simulink model "Induction_Machine_Model"  (Simulink 7.5)
settings: Solver=ode45  StartTime=0.0  StopTime=10.0  RelTol=1e-3
settings Model: Creator=CN  LastModifiedBy=pradhyumna
settings DebuggingCC: StrictBusMsg=Warning

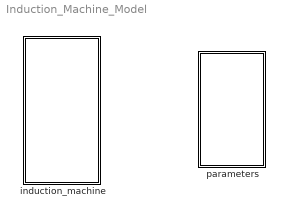
== system Induction_Machine_Model ==
  induction_machine : Subsystem
  parameters : Subsystem

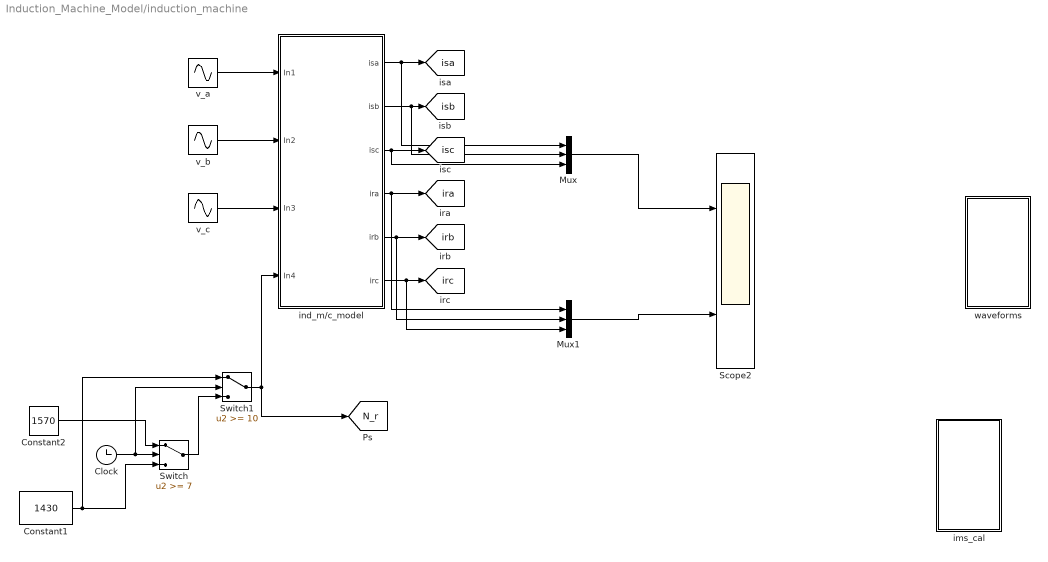
== system Induction_Machine_Model/induction_machine ==
  Clock : Clock
      settings: Decimation=10
  Constant1 : Constant  Value=1430  OutDataType=sfix(16)  OutScaling=2^0
  Constant2 : Constant  Value=1570  OutDataType=sfix(16)  OutScaling=2^0
  Mux : Mux  Inputs=3
  Mux1 : Mux  Inputs=3
  Scope2 : Scope  NumInputPorts=2
      settings: TimeRange=4.5  YMin=-30~-30  YMax=30~30  SampleInput=on  SampleTime=0.00001
  Switch : Switch  Threshold=7
  Switch1 : Switch  Threshold=10
  ims_cal : Subsystem
  ind_m/c_model : Subsystem
  v_a : Sin  Amplitude=239.6*sqrt(2)  Bias=0  Frequency=2*pi*50  Phase=0  Samples=10  SampleTime=0  Offset=0
  v_b : Sin  Amplitude=239.6*sqrt(2)  Bias=0  Frequency=2*pi*50  Phase=-2*pi/3  Samples=10  SampleTime=0  Offset=0
  v_c : Sin  Amplitude=239.6*sqrt(2)  Bias=0  Frequency=2*pi*50  Phase=-4*pi/3  Samples=10  SampleTime=0  Offset=0
  waveforms : Subsystem
  tag scope: N_r=global, ira=global, irb=global, irc=global, isa=global, isb=global, isc=global
  wires:
  ind_m/c_model/6(irc) -> [irc], Mux1/3
  ind_m/c_model/5(irb) -> [irb], Mux1/2
  ind_m/c_model/4(ira) -> [ira], Mux1/1
  ind_m/c_model/3(isc) -> [isc], Mux/3
  ind_m/c_model/2(isb) -> [isb], Mux/2
  ind_m/c_model/1(isa) -> [isa], Mux/1
  v_c/1 -> ind_m/c_model/3(In3)
  v_b/1 -> ind_m/c_model/2(In2)
  v_a/1 -> ind_m/c_model/1(In1)
  Mux/1 -> Scope2/1
  Mux1/1 -> Scope2/2
  Clock/1 -> Switch/2, Switch1/2
  Constant2/1 -> Switch/1
  Constant1/1 -> Switch/3, Switch1/1
  Switch/1 -> Switch1/3
  Switch1/1 -> ind_m/c_model/4(In4), [N_r]

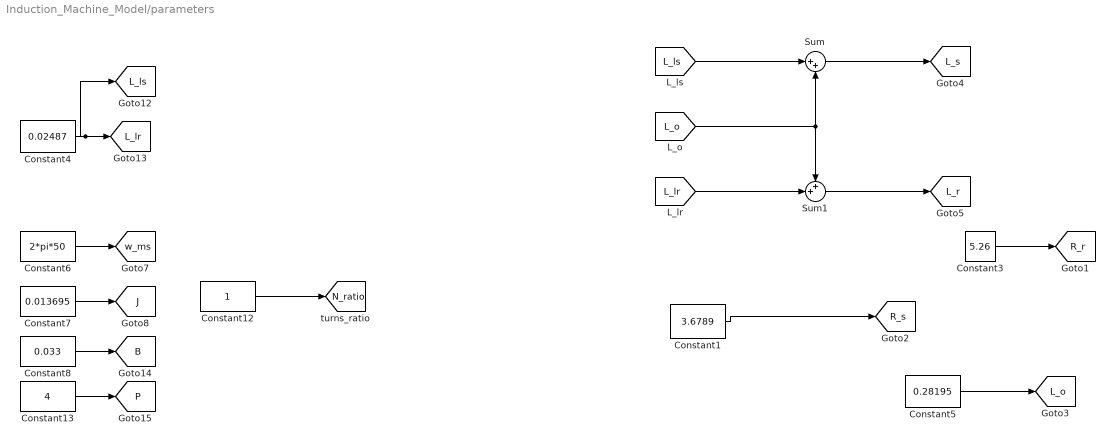
== system Induction_Machine_Model/parameters ==
  Constant1 : Constant  Value=3.6789  OutDataType=sfix(16)  OutScaling=2^0
  Constant12 : Constant  OutDataType=sfix(16)  OutScaling=2^0
  Constant13 : Constant  Value=4  OutDataType=sfix(16)  OutScaling=2^0
  Constant3 : Constant  Value=5.26  OutDataType=sfix(16)  OutScaling=2^0
  Constant4 : Constant  Value=0.02487  OutDataType=sfix(16)  OutScaling=2^0
  Constant5 : Constant  Value=0.28195  OutDataType=sfix(16)  OutScaling=2^0
  Constant6 : Constant  Value=2*pi*50  OutDataType=sfix(16)  OutScaling=2^0
  Constant7 : Constant  Value=0.013695  OutDataType=sfix(16)  OutScaling=2^0
  Constant8 : Constant  Value=0.033  OutDataType=sfix(16)  OutScaling=2^0
  Sum : Sum  Inputs=|++  OutDataType=sfix(16)  OutScaling=2^0
  Sum1 : Sum  Inputs=++|  OutDataType=sfix(16)  OutScaling=2^0
  tag scope: B=global, J=global, L_lr=global, L_ls=global, L_o=global, L_r=global, L_s=global, N_ratio=global, P=global, R_r=global, R_s=global, w_ms=global
  wires:
  Constant4/1 -> [L_lr], [L_ls]
  Constant6/1 -> [w_ms]
  Constant7/1 -> [J]
  Constant8/1 -> [B]
  Constant13/1 -> [P]
  Constant12/1 -> [N_ratio]
  [L_lr] -> Sum1/2
  [L_ls] -> Sum/1
  [L_o] -> Sum/2, Sum1/1
  Sum/1 -> [L_s]
  Sum1/1 -> [L_r]
  Constant3/1 -> [R_r]
  Constant5/1 -> [L_o]
  Constant1/1 -> [R_s]

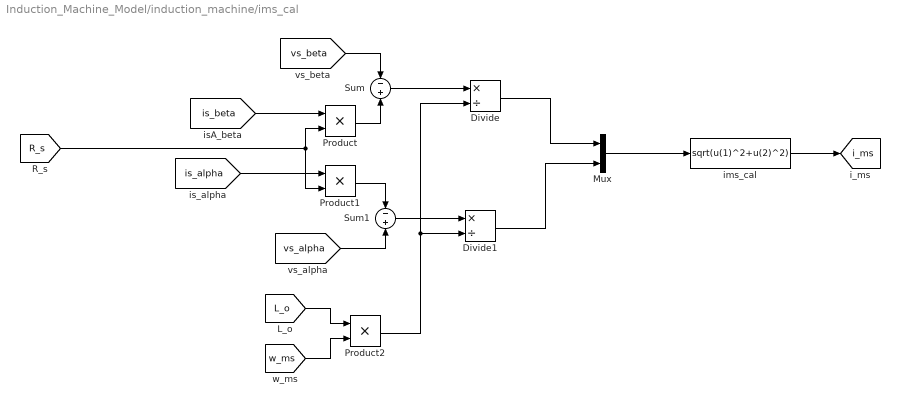
== system Induction_Machine_Model/induction_machine/ims_cal ==
  Divide : Product  Inputs=*/  OutDataType=sfix(16)  OutScaling=2^-10
  Divide1 : Product  Inputs=*/  OutDataType=sfix(16)  OutScaling=2^-10
  Mux : Mux  Inputs=2
  Product : Product  OutDataType=sfix(16)  OutScaling=2^0  RndMeth=Zero
  Product1 : Product  OutDataType=sfix(16)  OutScaling=2^0  RndMeth=Zero
  Product2 : Product  OutDataType=sfix(16)  OutScaling=2^0  RndMeth=Zero
  Sum : Sum  Inputs=-+  OutDataType=sfix(16)  OutScaling=2^0
  Sum1 : Sum  Inputs=-+  OutDataType=sfix(16)  OutScaling=2^0
  ims_cal : Fcn  Expr=sqrt(u(1)^2+u(2)^2)
  tag scope: i_ms=global
  wires:
  [is_beta] -> Product/1
  [is_alpha] -> Product1/1
  [R_s] -> Product/2, Product1/2
  [vs_beta] -> Sum/1
  Product/1 -> Sum/2
  Product1/1 -> Sum1/1
  [vs_alpha] -> Sum1/2
  [L_o] -> Product2/1
  [w_ms] -> Product2/2
  Sum/1 -> Divide/1
  Sum1/1 -> Divide1/1
  Product2/1 -> Divide/2, Divide1/2
  Divide/1 -> Mux/1
  Divide1/1 -> Mux/2
  Mux/1 -> ims_cal/1
  ims_cal/1 -> [i_ms]

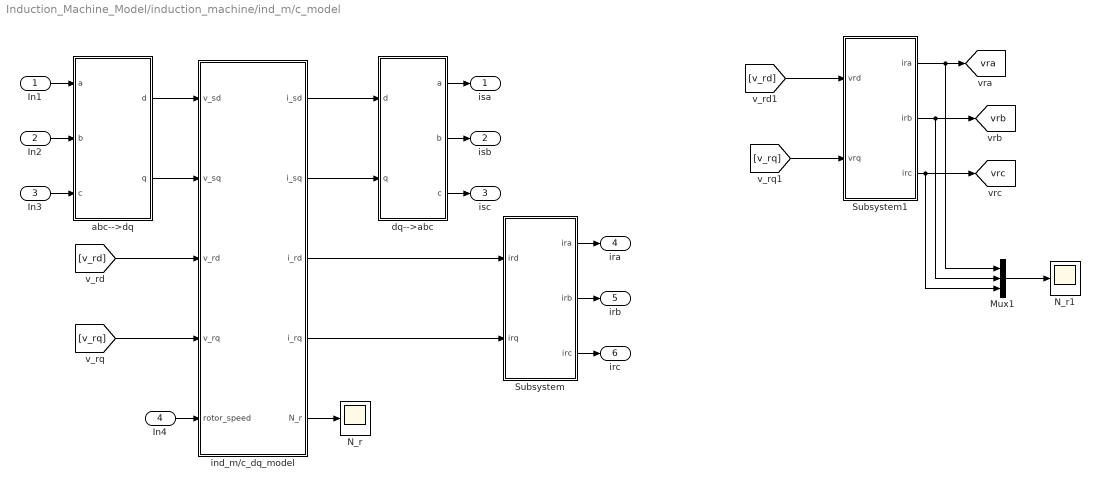
== system Induction_Machine_Model/induction_machine/ind_m/c_model ==
  In1 : Inport  OutDataType=sfix(16)  OutScaling=2^0
  In2 : Inport  Port=2  OutDataType=sfix(16)  OutScaling=2^0
  In3 : Inport  Port=3  OutDataType=sfix(16)  OutScaling=2^0
  In4 : Inport  Port=4  OutDataType=sfix(16)  OutScaling=2^0
  Mux1 : Mux  Inputs=3
  N_r : Scope
      settings: TimeRange=3  YMin=-7460  YMax=-7390  SaveName=ScopeData5  SampleInput=on  SampleTime=0.0001
  N_r1 : Scope
      settings: TimeRange=3  YMin=-7460  YMax=-7390  SaveName=ScopeData2  SampleInput=on  SampleTime=0.0001
  Subsystem : Subsystem
  Subsystem1 : Subsystem
  abc-->dq : Subsystem
  dq-->abc : Subsystem
  ind_m/c_dq_model : Subsystem
  isa : Outport  OutDataType=sfix(16)  OutScaling=2^0
  isb : Outport  Port=2  OutDataType=sfix(16)  OutScaling=2^0
  isc : Outport  Port=3  OutDataType=sfix(16)  OutScaling=2^0
  ira : Outport  Port=4  OutDataType=sfix(16)  OutScaling=2^0
  irb : Outport  Port=5  OutDataType=sfix(16)  OutScaling=2^0
  irc : Outport  Port=6  OutDataType=sfix(16)  OutScaling=2^0
  tag scope: vra=global, vrb=global, vrc=global
  wires:
  ind_m/c_dq_model/1(i_sd) -> dq-->abc/1(d)
  ind_m/c_dq_model/2(i_sq) -> dq-->abc/2(q)
  ind_m/c_dq_model/5(N_r) -> N_r/1
  abc-->dq/2(q) -> ind_m/c_dq_model/2(v_sq)
  abc-->dq/1(d) -> ind_m/c_dq_model/1(v_sd)
  ind_m/c_dq_model/3(i_rd) -> Subsystem/1(ird)
  ind_m/c_dq_model/4(i_rq) -> Subsystem/2(irq)
  In1/1 -> abc-->dq/1(a)
  dq-->abc/1(a) -> isa/1
  In2/1 -> abc-->dq/2(b)
  dq-->abc/2(b) -> isb/1
  In3/1 -> abc-->dq/3(c)
  dq-->abc/3(c) -> isc/1
  Subsystem/1(ira) -> ira/1
  Subsystem/2(irb) -> irb/1
  Subsystem/3(irc) -> irc/1
  In4/1 -> ind_m/c_dq_model/5(rotor_speed)
  [v_rd] -> ind_m/c_dq_model/3(v_rd)
  [v_rq] -> ind_m/c_dq_model/4(v_rq)
  [v_rd] -> Subsystem1/1(vrd)
  [v_rq] -> Subsystem1/2(vrq)
  Subsystem1/1(ira) -> [vra], Mux1/1
  Subsystem1/2(irb) -> [vrb], Mux1/2
  Subsystem1/3(irc) -> [vrc], Mux1/3
  Mux1/1 -> N_r1/1

== system Induction_Machine_Model/induction_machine/waveforms ==
  Mux : Mux  Inputs=3
  Mux1 : Mux  Inputs=3
  Mux2 : Mux  Inputs=3
  N_r : Scope  NumInputPorts=3
      settings: TimeRange=3  YMin=-7460~-5~-5  YMax=-7390~5~5  SampleInput=on  SampleTime=0.00001
  wires:
  [vsa] -> Mux/1
  [vsb] -> Mux/2
  [vsc] -> Mux/3
  [isa] -> Mux1/1
  [isb] -> Mux1/2
  [isc] -> Mux1/3
  [ira] -> Mux2/1
  [irb] -> Mux2/2
  [irc] -> Mux2/3
  Mux/1 -> N_r/1
  Mux1/1 -> N_r/2
  Mux2/1 -> N_r/3

== system Induction_Machine_Model/induction_machine/ind_m/c_model/Subsystem ==
  ird : Inport  OutDataType=sfix(16)  OutScaling=2^0
  irq : Inport  Port=2  OutDataType=sfix(16)  OutScaling=2^0
  ab-->abc : Subsystem
  dq-->ab : Subsystem
  ira : Outport  OutDataType=sfix(16)  OutScaling=2^0
  irb : Outport  Port=2  OutDataType=sfix(16)  OutScaling=2^0
  irc : Outport  Port=3  OutDataType=sfix(16)  OutScaling=2^0
  wires:
  dq-->ab/1(ir_a) -> ab-->abc/1(ir_a)
  dq-->ab/2(ir_b) -> ab-->abc/2(ir_b)
  ab-->abc/1(a) -> ira/1
  ird/1 -> dq-->ab/1(ird)
  ab-->abc/2(b) -> irb/1
  irq/1 -> dq-->ab/2(irq)
  ab-->abc/3(c) -> irc/1

== system Induction_Machine_Model/induction_machine/ind_m/c_model/Subsystem1 ==
  vrd : Inport  OutDataType=sfix(16)  OutScaling=2^0
  vrq : Inport  Port=2  OutDataType=sfix(16)  OutScaling=2^0
  ab-->abc : Subsystem
  dq-->ab : Subsystem
  ira : Outport  OutDataType=sfix(16)  OutScaling=2^0
  irb : Outport  Port=2  OutDataType=sfix(16)  OutScaling=2^0
  irc : Outport  Port=3  OutDataType=sfix(16)  OutScaling=2^0
  wires:
  ab-->abc/3(c) -> irc/1
  vrq/1 -> dq-->ab/2(vrq)
  ab-->abc/2(b) -> irb/1
  vrd/1 -> dq-->ab/1(vrd)
  ab-->abc/1(a) -> ira/1
  dq-->ab/2(ir_b) -> ab-->abc/2(ir_b)
  dq-->ab/1(ir_a) -> ab-->abc/1(ir_a)

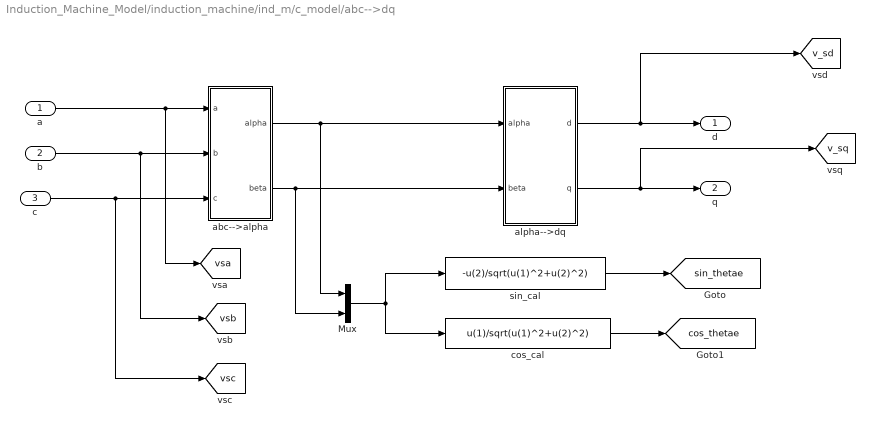
== system Induction_Machine_Model/induction_machine/ind_m/c_model/abc-->dq ==
  a : Inport  OutDataType=sfix(16)  OutScaling=2^0
  b : Inport  Port=2  OutDataType=sfix(16)  OutScaling=2^0
  c : Inport  Port=3  OutDataType=sfix(16)  OutScaling=2^0
  Mux : Mux  Inputs=2
  abc-->alpha : Subsystem
  alpha-->dq : Subsystem
  cos_cal : Fcn  Expr=u(1)/sqrt(u(1)^2+u(2)^2)
  sin_cal : Fcn  Expr=-u(2)/sqrt(u(1)^2+u(2)^2)
  d : Outport  OutDataType=sfix(16)  OutScaling=2^0
  q : Outport  Port=2  OutDataType=sfix(16)  OutScaling=2^0
  tag scope: cos_thetae=global, sin_thetae=global, v_sd=global, v_sq=global, vsa=global, vsb=global, vsc=global
  wires:
  abc-->alpha/1(alpha) -> alpha-->dq/1(alpha), Mux/1
  abc-->alpha/2(beta) -> alpha-->dq/2(beta), Mux/2
  a/1 -> abc-->alpha/1(a), [vsa]
  alpha-->dq/1(d) -> d/1, [v_sd]
  b/1 -> abc-->alpha/2(b), [vsb]
  alpha-->dq/2(q) -> q/1, [v_sq]
  c/1 -> abc-->alpha/3(c), [vsc]
  Mux/1 -> sin_cal/1, cos_cal/1
  sin_cal/1 -> [sin_thetae]
  cos_cal/1 -> [cos_thetae]

== system Induction_Machine_Model/induction_machine/ind_m/c_model/dq-->abc ==
  d : Inport  OutDataType=sfix(16)  OutScaling=2^0
  q : Inport  Port=2  OutDataType=sfix(16)  OutScaling=2^0
  alpha-->abc : Subsystem
  dq-->alpha : Subsystem
  a : Outport  OutDataType=sfix(16)  OutScaling=2^0
  b : Outport  Port=2  OutDataType=sfix(16)  OutScaling=2^0
  c : Outport  Port=3  OutDataType=sfix(16)  OutScaling=2^0
  wires:
  dq-->alpha/1(alpha) -> alpha-->abc/1(alpha)
  dq-->alpha/2(beta) -> alpha-->abc/2(beta)
  alpha-->abc/1(a) -> a/1
  d/1 -> dq-->alpha/1(d)
  alpha-->abc/2(b) -> b/1
  q/1 -> dq-->alpha/2(q)
  alpha-->abc/3(c) -> c/1

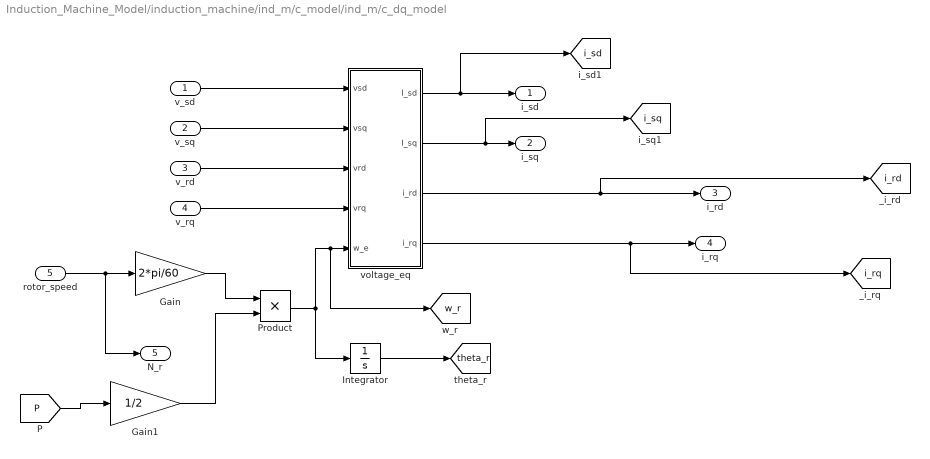
== system Induction_Machine_Model/induction_machine/ind_m/c_model/ind_m/c_dq_model ==
  v_sd : Inport  OutDataType=sfix(16)  OutScaling=2^0
  v_sq : Inport  Port=2  OutDataType=sfix(16)  OutScaling=2^0
  v_rd : Inport  Port=3  OutDataType=sfix(16)  OutScaling=2^0
  v_rq : Inport  Port=4  OutDataType=sfix(16)  OutScaling=2^0
  rotor_speed : Inport  Port=5  OutDataType=sfix(16)  OutScaling=2^0
  Gain : Gain  Gain=2*pi/60  ParameterDataType=sfix(16)  ParameterScaling=2^0  OutDataType=sfix(16)  OutScaling=2^0
  Gain1 : Gain  Gain=1/2  ParameterDataType=sfix(16)  ParameterScaling=2^0  OutDataType=sfix(16)  OutScaling=2^0
  Integrator : Integrator
  Product : Product  OutDataType=sfix(16)  OutScaling=2^0  RndMeth=Zero
  voltage_eq : Subsystem
  i_sd : Outport  OutDataType=sfix(16)  OutScaling=2^0
  i_sq : Outport  Port=2  OutDataType=sfix(16)  OutScaling=2^0
  i_rd : Outport  Port=3  OutDataType=sfix(16)  OutScaling=2^0
  i_rq : Outport  Port=4  OutDataType=sfix(16)  OutScaling=2^0
  N_r : Outport  Port=5  OutDataType=sfix(16)  OutScaling=2^0
  tag scope: i_rd=global, i_rq=global, i_sd=global, i_sq=global, theta_r=global, w_r=global
  wires:
  v_sd/1 -> voltage_eq/1(vsd)
  v_sq/1 -> voltage_eq/2(vsq)
  v_rd/1 -> voltage_eq/3(vrd)
  v_rq/1 -> voltage_eq/4(vrq)
  voltage_eq/1(I_sd) -> i_sd/1, [i_sd]
  voltage_eq/2(I_sq) -> i_sq/1, [i_sq]
  voltage_eq/3(i_rd) -> i_rd/1, [i_rd]
  voltage_eq/4(i_rq) -> i_rq/1, [i_rq]
  rotor_speed/1 -> Gain/1, N_r/1
  Gain/1 -> Product/1
  [P] -> Gain1/1
  Gain1/1 -> Product/2
  Product/1 -> Integrator/1, voltage_eq/5(w_e), [w_r]
  Integrator/1 -> [theta_r]

== system Induction_Machine_Model/induction_machine/ind_m/c_model/Subsystem/ab-->abc ==
  ir_a : Inport  OutDataType=sfix(16)  OutScaling=2^0
  ir_b : Inport  Port=2  OutDataType=sfix(16)  OutScaling=2^0
  Fcn : Fcn  Expr=u(1)
  Fcn1 : Fcn  Expr=-u(1)/2-u(2)*sqrt(3)/2
  Fcn2 : Fcn  Expr=-u(1)/2+u(2)*sqrt(3)/2
  Mux : Mux  Inputs=2
  a : Outport  OutDataType=sfix(16)  OutScaling=2^0
  b : Outport  Port=2  OutDataType=sfix(16)  OutScaling=2^0
  c : Outport  Port=3  OutDataType=sfix(16)  OutScaling=2^0
  wires:
  Mux/1 -> Fcn/1, Fcn1/1, Fcn2/1
  Fcn/1 -> a/1
  Fcn1/1 -> b/1
  Fcn2/1 -> c/1
  ir_a/1 -> Mux/1
  ir_b/1 -> Mux/2

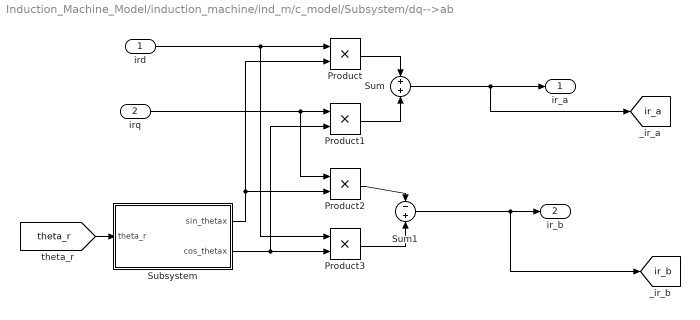
== system Induction_Machine_Model/induction_machine/ind_m/c_model/Subsystem/dq-->ab ==
  ird : Inport  OutDataType=sfix(16)  OutScaling=2^0
  irq : Inport  Port=2  OutDataType=sfix(16)  OutScaling=2^0
  Product{,1..3} (4 alike) : Product  OutDataType=sfix(16)  OutScaling=2^0  RndMeth=Zero
  Subsystem : Subsystem
  Sum : Sum  OutDataType=sfix(16)  OutScaling=2^0
  Sum1 : Sum  Inputs=-+  OutDataType=sfix(16)  OutScaling=2^0
  ir_a : Outport  OutDataType=sfix(16)  OutScaling=2^0
  ir_b : Outport  Port=2  OutDataType=sfix(16)  OutScaling=2^0
  tag scope: ir_a=global, ir_b=global
  wires:
  [theta_r] -> Subsystem/1(theta_r)
  ird/1 -> Product3/1, Product/1
  Subsystem/1(sin_thetax) -> Product/2, Product2/2
  irq/1 -> Product2/1, Product1/1
  Subsystem/2(cos_thetax) -> Product1/2, Product3/2
  Product/1 -> Sum/1
  Product1/1 -> Sum/2
  Product2/1 -> Sum1/1
  Product3/1 -> Sum1/2
  Sum/1 -> ir_a/1, [ir_a]
  Sum1/1 -> ir_b/1, [ir_b]

== system Induction_Machine_Model/induction_machine/ind_m/c_model/Subsystem1/ab-->abc ==
  ir_a : Inport  OutDataType=sfix(16)  OutScaling=2^0
  ir_b : Inport  Port=2  OutDataType=sfix(16)  OutScaling=2^0
  Fcn : Fcn  Expr=u(1)
  Fcn1 : Fcn  Expr=-u(1)/2-u(2)*sqrt(3)/2
  Fcn2 : Fcn  Expr=-u(1)/2+u(2)*sqrt(3)/2
  Mux : Mux  Inputs=2
  a : Outport  OutDataType=sfix(16)  OutScaling=2^0
  b : Outport  Port=2  OutDataType=sfix(16)  OutScaling=2^0
  c : Outport  Port=3  OutDataType=sfix(16)  OutScaling=2^0
  wires:
  ir_b/1 -> Mux/2
  ir_a/1 -> Mux/1
  Fcn2/1 -> c/1
  Fcn1/1 -> b/1
  Fcn/1 -> a/1
  Mux/1 -> Fcn2/1, Fcn1/1, Fcn/1

== system Induction_Machine_Model/induction_machine/ind_m/c_model/Subsystem1/dq-->ab ==
  vrd : Inport  OutDataType=sfix(16)  OutScaling=2^0
  vrq : Inport  Port=2  OutDataType=sfix(16)  OutScaling=2^0
  Product{,1..3} (4 alike) : Product  OutDataType=sfix(16)  OutScaling=2^0  RndMeth=Zero
  Subsystem : Subsystem
  Sum : Sum  OutDataType=sfix(16)  OutScaling=2^0
  Sum1 : Sum  Inputs=-+  OutDataType=sfix(16)  OutScaling=2^0
  ir_a : Outport  OutDataType=sfix(16)  OutScaling=2^0
  ir_b : Outport  Port=2  OutDataType=sfix(16)  OutScaling=2^0
  wires:
  Sum1/1 -> ir_b/1
  Sum/1 -> ir_a/1
  Product3/1 -> Sum1/2
  Product2/1 -> Sum1/1
  Product1/1 -> Sum/2
  Product/1 -> Sum/1
  Subsystem/2(cos_thetax) -> Product3/2, Product1/2
  vrq/1 -> Product1/1, Product2/1
  Subsystem/1(sin_thetax) -> Product2/2, Product/2
  vrd/1 -> Product/1, Product3/1
  [theta_r] -> Subsystem/1(theta_r)

== system Induction_Machine_Model/induction_machine/ind_m/c_model/abc-->dq/abc-->alpha ==
  a : Inport  OutDataType=sfix(16)  OutScaling=2^0
  b : Inport  Port=2  OutDataType=sfix(16)  OutScaling=2^0
  c : Inport  Port=3  OutDataType=sfix(16)  OutScaling=2^0
  Mux : Mux  Inputs=3
  alpha_cal : Fcn  Expr=2/3*(u(1)+u(2)*cos(-2*pi/3)+u(3)*cos(-4*pi/3))
  beta_cal : Fcn  Expr=2/3*(u(2)*sin(-2*pi/3)+u(3)*sin(-4*pi/3))
  alpha : Outport  OutDataType=sfix(16)  OutScaling=2^0
  beta : Outport  Port=2  OutDataType=sfix(16)  OutScaling=2^0
  tag scope: vs_alpha=global, vs_beta=global
  wires:
  Mux/1 -> alpha_cal/1, beta_cal/1
  a/1 -> Mux/1
  alpha_cal/1 -> alpha/1, [vs_alpha]
  b/1 -> Mux/2
  beta_cal/1 -> beta/1, [vs_beta]
  c/1 -> Mux/3

== system Induction_Machine_Model/induction_machine/ind_m/c_model/abc-->dq/alpha-->dq ==
  alpha : Inport  OutDataType=sfix(16)  OutScaling=2^0
  beta : Inport  Port=2  OutDataType=sfix(16)  OutScaling=2^0
  Product{1..4} (4 alike) : Product  OutDataType=sfix(16)  OutScaling=2^0  RndMeth=Zero
  Sum : Sum  OutDataType=sfix(16)  OutScaling=2^0
  Sum1 : Sum  Inputs=+-  OutDataType=sfix(16)  OutScaling=2^0
  d : Outport  OutDataType=sfix(16)  OutScaling=2^0
  q : Outport  Port=2  OutDataType=sfix(16)  OutScaling=2^0
  wires:
  alpha/1 -> Product3/1, Product1/1
  beta/1 -> Product4/1, Product2/1
  [cos_thetae] -> Product3/2, Product2/2
  [sin_thetae] -> Product4/2, Product1/2
  Product1/1 -> Sum/1
  Product2/1 -> Sum/2
  Product3/1 -> Sum1/1
  Product4/1 -> Sum1/2
  Sum/1 -> d/1
  Sum1/1 -> q/1

== system Induction_Machine_Model/induction_machine/ind_m/c_model/dq-->abc/alpha-->abc ==
  alpha : Inport  OutDataType=sfix(16)  OutScaling=2^0
  beta : Inport  Port=2  OutDataType=sfix(16)  OutScaling=2^0
  Fcn : Fcn  Expr=u(1)
  Fcn1 : Fcn  Expr=-u(1)/2-u(2)*sqrt(3)/2
  Fcn2 : Fcn  Expr=-u(1)/2+u(2)*sqrt(3)/2
  Mux : Mux  Inputs=2
  a : Outport  OutDataType=sfix(16)  OutScaling=2^0
  b : Outport  Port=2  OutDataType=sfix(16)  OutScaling=2^0
  c : Outport  Port=3  OutDataType=sfix(16)  OutScaling=2^0
  wires:
  Mux/1 -> Fcn/1, Fcn1/1, Fcn2/1
  Fcn/1 -> a/1
  Fcn1/1 -> b/1
  Fcn2/1 -> c/1
  alpha/1 -> Mux/1
  beta/1 -> Mux/2

== system Induction_Machine_Model/induction_machine/ind_m/c_model/dq-->abc/dq-->alpha ==
  d : Inport  OutDataType=sfix(16)  OutScaling=2^0
  q : Inport  Port=2  OutDataType=sfix(16)  OutScaling=2^0
  Product{1..4} (4 alike) : Product  OutDataType=sfix(16)  OutScaling=2^0  RndMeth=Zero
  Sum : Sum  OutDataType=sfix(16)  OutScaling=2^0
  Sum1 : Sum  Inputs=+-  OutDataType=sfix(16)  OutScaling=2^0
  alpha : Outport  OutDataType=sfix(16)  OutScaling=2^0
  beta : Outport  Port=2  OutDataType=sfix(16)  OutScaling=2^0
  tag scope: is_alpha=global, is_beta=global
  wires:
  d/1 -> Product1/1, Product3/1
  q/1 -> Product2/1, Product4/1
  [cos_thetae] -> Product3/2, Product2/2
  [sin_thetae] -> Product4/2, Product1/2
  Product1/1 -> Sum/1
  Product2/1 -> Sum/2
  Product3/1 -> Sum1/1
  Product4/1 -> Sum1/2
  Sum/1 -> alpha/1, [is_alpha]
  Sum1/1 -> beta/1, [is_beta]

== system Induction_Machine_Model/induction_machine/ind_m/c_model/ind_m/c_dq_model/voltage_eq ==
  vsd : Inport  OutDataType=sfix(16)  OutScaling=2^0
  vsq : Inport  Port=2  OutDataType=sfix(16)  OutScaling=2^0
  vrd : Inport  Port=3  OutDataType=sfix(16)  OutScaling=2^0
  vrq : Inport  Port=4  OutDataType=sfix(16)  OutScaling=2^0
  w_e : Inport  Port=5  OutDataType=sfix(16)  OutScaling=2^0
  rotor_d_eq : Subsystem
  rotor_q_eq : Subsystem
  stator_d_eq : Subsystem
  stator_q_eq : Subsystem
  I_sd : Outport  OutDataType=sfix(16)  OutScaling=2^0
  I_sq : Outport  Port=2  OutDataType=sfix(16)  OutScaling=2^0
  i_rd : Outport  Port=3  OutDataType=sfix(16)  OutScaling=2^0
  i_rq : Outport  Port=4  OutDataType=sfix(16)  OutScaling=2^0
  wires:
  stator_d_eq/1(i_sd) -> rotor_q_eq/2(isd), rotor_d_eq/2(isd), stator_q_eq/2(isd), stator_d_eq/2(isd), I_sd/1
  stator_q_eq/1(i_sq) -> stator_d_eq/3(isq), rotor_q_eq/3(isq), rotor_d_eq/3(isq), stator_q_eq/3(isq), I_sq/1
  rotor_d_eq/1(i_rd) -> stator_d_eq/4("ird\""), stator_q_eq/4("ird\""), rotor_q_eq/4("ird\""), rotor_d_eq/4("ird\""), i_rd/1
  rotor_q_eq/1(i_rq) -> stator_d_eq/5("irq\""), stator_q_eq/5("irq\""), rotor_d_eq/5("irq\""), rotor_q_eq/5("irq\""), i_rq/1
  w_e/1 -> rotor_q_eq/6(w_e), rotor_d_eq/6(w_e)
  vsd/1 -> stator_d_eq/1(v_sd)
  vsq/1 -> stator_q_eq/1(v_sq)
  vrd/1 -> rotor_d_eq/1(v_rd)
  vrq/1 -> rotor_q_eq/1(v_rq)

== system Induction_Machine_Model/induction_machine/ind_m/c_model/Subsystem/dq-->ab/Subsystem ==
  theta_r : Inport  OutDataType=sfix(16)  OutScaling=2^0
  Product{,1..3} (4 alike) : Product  OutDataType=sfix(16)  OutScaling=2^0  RndMeth=Zero
  Sum : Sum  Inputs=+-  OutDataType=sfix(16)  OutScaling=2^0
  Sum1 : Sum  OutDataType=sfix(16)  OutScaling=2^0
  cos_thetar : Trigonometry  Operator=cos
  sin_thetar : Trigonometry
  sin_thetax : Outport  OutDataType=sfix(16)  OutScaling=2^0
  cos_thetax : Outport  Port=2  OutDataType=sfix(16)  OutScaling=2^0
  wires:
  theta_r/1 -> cos_thetar/1, sin_thetar/1
  [sin_thetae] -> Product/1, Product2/1
  cos_thetar/1 -> Product/2, Product3/2
  [cos_thetae] -> Product1/1, Product3/1
  sin_thetar/1 -> Product1/2, Product2/2
  Product/1 -> Sum/1
  Product1/1 -> Sum/2
  Product2/1 -> Sum1/1
  Product3/1 -> Sum1/2
  Sum/1 -> sin_thetax/1
  Sum1/1 -> cos_thetax/1

== system Induction_Machine_Model/induction_machine/ind_m/c_model/Subsystem1/dq-->ab/Subsystem ==
  theta_r : Inport  OutDataType=sfix(16)  OutScaling=2^0
  Product{,1..3} (4 alike) : Product  OutDataType=sfix(16)  OutScaling=2^0  RndMeth=Zero
  Sum : Sum  Inputs=+-  OutDataType=sfix(16)  OutScaling=2^0
  Sum1 : Sum  OutDataType=sfix(16)  OutScaling=2^0
  cos_thetar : Trigonometry  Operator=cos
  sin_thetar : Trigonometry
  sin_thetax : Outport  OutDataType=sfix(16)  OutScaling=2^0
  cos_thetax : Outport  Port=2  OutDataType=sfix(16)  OutScaling=2^0
  wires:
  Sum1/1 -> cos_thetax/1
  Sum/1 -> sin_thetax/1
  Product3/1 -> Sum1/2
  Product2/1 -> Sum1/1
  Product1/1 -> Sum/2
  Product/1 -> Sum/1
  sin_thetar/1 -> Product2/2, Product1/2
  [cos_thetae] -> Product3/1, Product1/1
  cos_thetar/1 -> Product3/2, Product/2
  [sin_thetae] -> Product2/1, Product/1
  theta_r/1 -> sin_thetar/1, cos_thetar/1

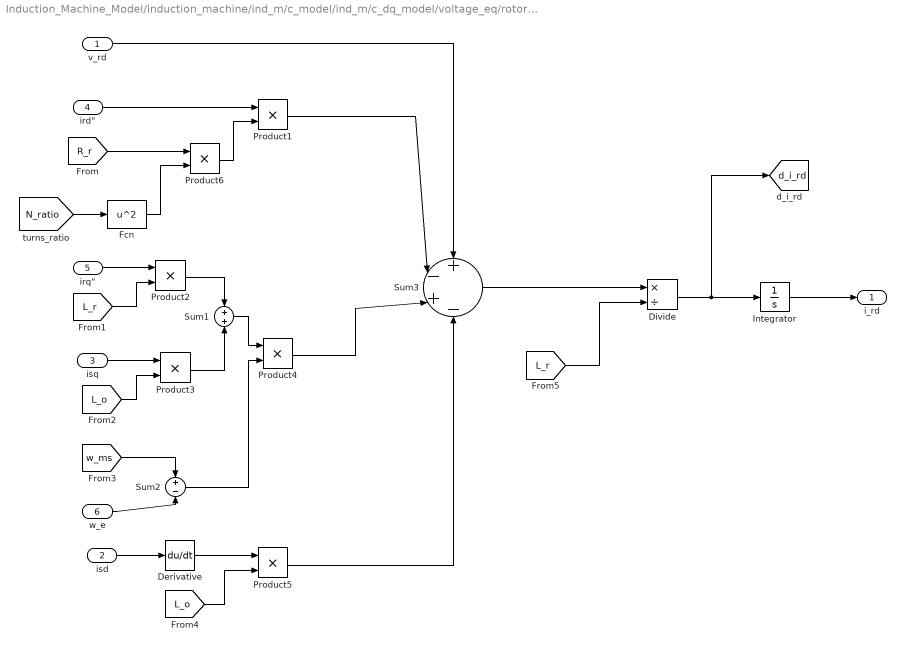
== system Induction_Machine_Model/induction_machine/ind_m/c_model/ind_m/c_dq_model/voltage_eq/rotor_d_eq ==
  v_rd : Inport  OutDataType=sfix(16)  OutScaling=2^0
  isd : Inport  Port=2  OutDataType=sfix(16)  OutScaling=2^0
  isq : Inport  Port=3  OutDataType=sfix(16)  OutScaling=2^0
  "ird\"" : Inport  Port=4  OutDataType=sfix(16)  OutScaling=2^0
  "irq\"" : Inport  Port=5  OutDataType=sfix(16)  OutScaling=2^0
  w_e : Inport  Port=6  OutDataType=sfix(16)  OutScaling=2^0
  Derivative : Derivative
  Divide : Product  Inputs=*/  OutDataType=sfix(16)  OutScaling=2^-10
  Fcn : Fcn  Expr=u^2
  Integrator : Integrator
  Product{1..6} (6 alike) : Product  OutDataType=sfix(16)  OutScaling=2^0  RndMeth=Zero
  Sum1 : Sum  OutDataType=sfix(16)  OutScaling=2^0
  Sum2 : Sum  Inputs=+-  OutDataType=sfix(16)  OutScaling=2^0
  Sum3 : Sum  Inputs=+-+-  OutDataType=sfix(16)  OutScaling=2^0
  i_rd : Outport  OutDataType=sfix(16)  OutScaling=2^0
  tag scope: d_i_rd=global
  wires:
  "ird\""/1 -> Product1/1
  "irq\""/1 -> Product2/1
  [L_r] -> Product2/2
  isq/1 -> Product3/1
  [L_o] -> Product3/2
  Product2/1 -> Sum1/1
  Product3/1 -> Sum1/2
  [w_ms] -> Sum2/1
  w_e/1 -> Sum2/2
  Sum1/1 -> Product4/1
  Sum2/1 -> Product4/2
  isd/1 -> Derivative/1
  Derivative/1 -> Product5/1
  [L_o] -> Product5/2
  v_rd/1 -> Sum3/1
  Product1/1 -> Sum3/2
  Product4/1 -> Sum3/3
  Product5/1 -> Sum3/4
  Sum3/1 -> Divide/1
  [L_r] -> Divide/2
  Divide/1 -> [d_i_rd], Integrator/1
  [N_ratio] -> Fcn/1
  [R_r] -> Product6/1
  Fcn/1 -> Product6/2
  Product6/1 -> Product1/2
  Integrator/1 -> i_rd/1

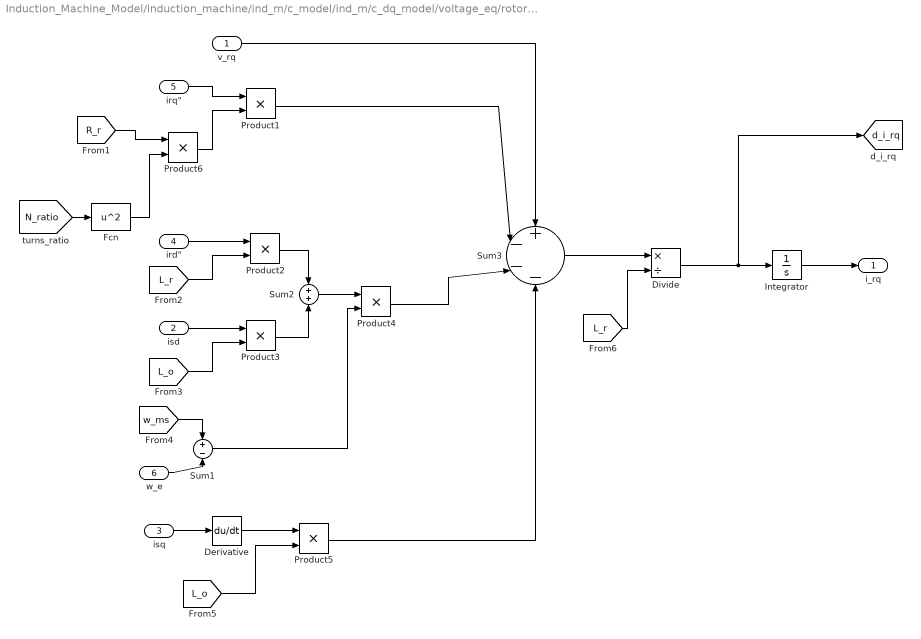
== system Induction_Machine_Model/induction_machine/ind_m/c_model/ind_m/c_dq_model/voltage_eq/rotor_q_eq ==
  v_rq : Inport  OutDataType=sfix(16)  OutScaling=2^0
  isd : Inport  Port=2  OutDataType=sfix(16)  OutScaling=2^0
  isq : Inport  Port=3  OutDataType=sfix(16)  OutScaling=2^0
  "ird\"" : Inport  Port=4  OutDataType=sfix(16)  OutScaling=2^0
  "irq\"" : Inport  Port=5  OutDataType=sfix(16)  OutScaling=2^0
  w_e : Inport  Port=6  OutDataType=sfix(16)  OutScaling=2^0
  Derivative : Derivative
  Divide : Product  Inputs=*/  OutDataType=sfix(16)  OutScaling=2^-10
  Fcn : Fcn  Expr=u^2
  Integrator : Integrator
  Product{1..6} (6 alike) : Product  OutDataType=sfix(16)  OutScaling=2^0  RndMeth=Zero
  Sum1 : Sum  Inputs=+-  OutDataType=sfix(16)  OutScaling=2^0
  Sum2 : Sum  OutDataType=sfix(16)  OutScaling=2^0
  Sum3 : Sum  Inputs=+---  OutDataType=sfix(16)  OutScaling=2^0
  i_rq : Outport  OutDataType=sfix(16)  OutScaling=2^0
  tag scope: d_i_rq=global
  wires:
  "irq\""/1 -> Product1/1
  Product6/1 -> Product1/2
  "ird\""/1 -> Product2/1
  [L_r] -> Product2/2
  isd/1 -> Product3/1
  [L_o] -> Product3/2
  [w_ms] -> Sum1/1
  w_e/1 -> Sum1/2
  Product2/1 -> Sum2/1
  Product3/1 -> Sum2/2
  Sum2/1 -> Product4/1
  Sum1/1 -> Product4/2
  isq/1 -> Derivative/1
  Derivative/1 -> Product5/1
  [L_o] -> Product5/2
  v_rq/1 -> Sum3/1
  Product1/1 -> Sum3/2
  Product4/1 -> Sum3/3
  Product5/1 -> Sum3/4
  Sum3/1 -> Divide/1
  [L_r] -> Divide/2
  Divide/1 -> [d_i_rq], Integrator/1
  [N_ratio] -> Fcn/1
  [R_r] -> Product6/1
  Fcn/1 -> Product6/2
  Integrator/1 -> i_rq/1

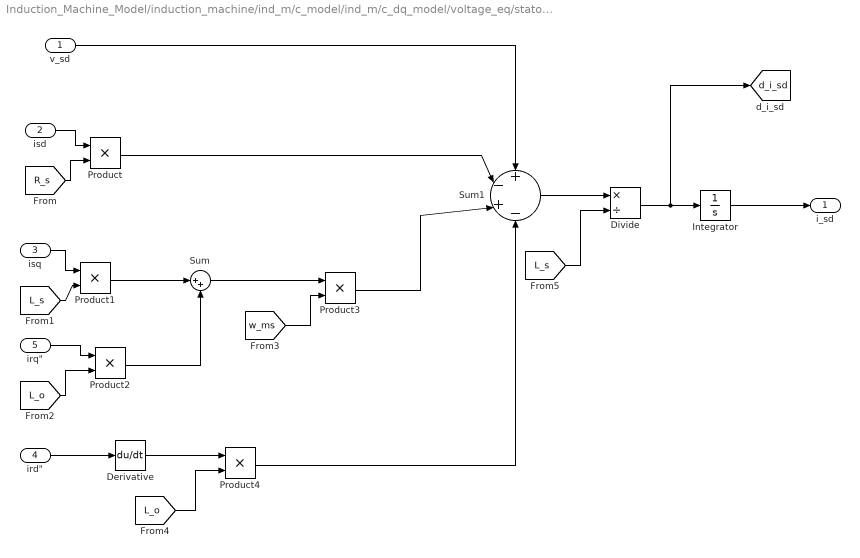
== system Induction_Machine_Model/induction_machine/ind_m/c_model/ind_m/c_dq_model/voltage_eq/stator_d_eq ==
  v_sd : Inport  OutDataType=sfix(16)  OutScaling=2^0
  isd : Inport  Port=2  OutDataType=sfix(16)  OutScaling=2^0
  isq : Inport  Port=3  OutDataType=sfix(16)  OutScaling=2^0
  "ird\"" : Inport  Port=4  OutDataType=sfix(16)  OutScaling=2^0
  "irq\"" : Inport  Port=5  OutDataType=sfix(16)  OutScaling=2^0
  Derivative : Derivative
  Divide : Product  Inputs=*/  OutDataType=sfix(16)  OutScaling=2^-10
  Integrator : Integrator
  Product{,1..4} (5 alike) : Product  OutDataType=sfix(16)  OutScaling=2^0  RndMeth=Zero
  Sum : Sum  Inputs=|++  OutDataType=sfix(16)  OutScaling=2^0
  Sum1 : Sum  Inputs=+-+-  OutDataType=sfix(16)  OutScaling=2^0
  i_sd : Outport  OutDataType=sfix(16)  OutScaling=2^0
  tag scope: d_i_sd=global
  wires:
  isd/1 -> Product/1
  [R_s] -> Product/2
  isq/1 -> Product1/1
  [L_s] -> Product1/2
  "irq\""/1 -> Product2/1
  [L_o] -> Product2/2
  Product1/1 -> Sum/1
  Product2/1 -> Sum/2
  [w_ms] -> Product3/2
  Sum/1 -> Product3/1
  "ird\""/1 -> Derivative/1
  Derivative/1 -> Product4/1
  [L_o] -> Product4/2
  v_sd/1 -> Sum1/1
  Product/1 -> Sum1/2
  Product3/1 -> Sum1/3
  Product4/1 -> Sum1/4
  Sum1/1 -> Divide/1
  [L_s] -> Divide/2
  Divide/1 -> Integrator/1, [d_i_sd]
  Integrator/1 -> i_sd/1

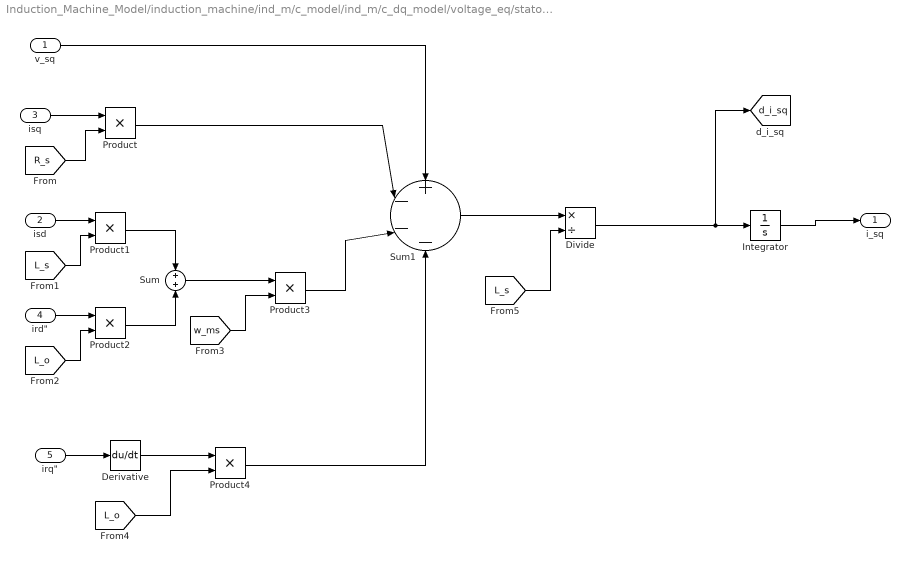
== system Induction_Machine_Model/induction_machine/ind_m/c_model/ind_m/c_dq_model/voltage_eq/stator_q_eq ==
  v_sq : Inport  OutDataType=sfix(16)  OutScaling=2^0
  isd : Inport  Port=2  OutDataType=sfix(16)  OutScaling=2^0
  isq : Inport  Port=3  OutDataType=sfix(16)  OutScaling=2^0
  "ird\"" : Inport  Port=4  OutDataType=sfix(16)  OutScaling=2^0
  "irq\"" : Inport  Port=5  OutDataType=sfix(16)  OutScaling=2^0
  Derivative : Derivative
  Divide : Product  Inputs=*/  OutDataType=sfix(16)  OutScaling=2^-10
  Integrator : Integrator
  Product{,1..4} (5 alike) : Product  OutDataType=sfix(16)  OutScaling=2^0  RndMeth=Zero
  Sum : Sum  OutDataType=sfix(16)  OutScaling=2^0
  Sum1 : Sum  Inputs=+---  OutDataType=sfix(16)  OutScaling=2^0
  i_sq : Outport  OutDataType=sfix(16)  OutScaling=2^0
  tag scope: d_i_sq=global
  wires:
  isq/1 -> Product/1
  [R_s] -> Product/2
  isd/1 -> Product1/1
  [L_s] -> Product1/2
  "ird\""/1 -> Product2/1
  [L_o] -> Product2/2
  Product1/1 -> Sum/1
  Product2/1 -> Sum/2
  Sum/1 -> Product3/1
  [w_ms] -> Product3/2
  "irq\""/1 -> Derivative/1
  Derivative/1 -> Product4/1
  [L_o] -> Product4/2
  v_sq/1 -> Sum1/1
  Product/1 -> Sum1/2
  Product3/1 -> Sum1/3
  Product4/1 -> Sum1/4
  Sum1/1 -> Divide/1
  [L_s] -> Divide/2
  Divide/1 -> [d_i_sq], Integrator/1
  Integrator/1 -> i_sq/1
